simulink model "SWC_CGW_type"  (R2021b)
settings: Solver=FixedStepDiscrete  StartTime=0.0  StopTime=10.0  RelTol=1e-3
(part 3 of 3)

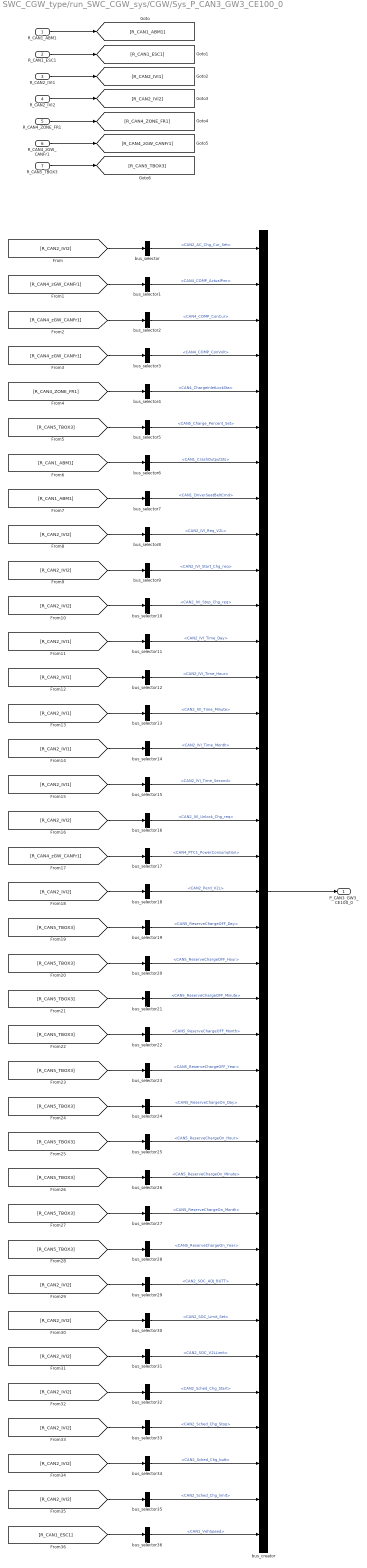
== system SWC_CGW_type/run_SWC_CGW_sys/CGW/Sys_P_CAN3_GW3_CE100_0 ==
  R_CAN1_ABM1 : Inport
  R_CAN1_ESC1 : Inport  Port=2
  R_CAN2_IVI1 : Inport  Port=3
  R_CAN2_IVI2 : Inport  Port=4
  R_CAN4_ZONE_FR1 : Inport  Port=5
  R_CAN4_zGW_CANFr1 : Inport  Port=6
  R_CAN5_TBOX3 : Inport  Port=7
  bus_creator : BusCreator  Inputs=37  OutDataTypeStr=Bus: DT_CAN3_SG_GW3_CE100_0  NonVirtualBus=on
  bus_selector : BusSelector  OutputSignals=CAN2_AC_Chg_Cur_Set
  bus_selector1 : BusSelector  OutputSignals=CAN4_COMP_ActualPwr
  bus_selector10 : BusSelector  OutputSignals=CAN2_IVI_Stop_Chg_req
  bus_selector11 : BusSelector  OutputSignals=CAN2_IVI_Time_Day
  bus_selector12 : BusSelector  OutputSignals=CAN2_IVI_Time_Hour
  bus_selector13 : BusSelector  OutputSignals=CAN2_IVI_Time_Minute
  bus_selector14 : BusSelector  OutputSignals=CAN2_IVI_Time_Month
  bus_selector15 : BusSelector  OutputSignals=CAN2_IVI_Time_Second
  bus_selector16 : BusSelector  OutputSignals=CAN2_IVI_Unlock_Chg_req
  bus_selector17 : BusSelector  OutputSignals=CAN4_PTC1_PowerConsumption
  bus_selector18 : BusSelector  OutputSignals=CAN2_Perd_V2L
  bus_selector19 : BusSelector  OutputSignals=CAN5_ReserveChargeOFF_Day
  bus_selector2 : BusSelector  OutputSignals=CAN4_COMP_ConCur
  bus_selector20 : BusSelector  OutputSignals=CAN5_ReserveChargeOFF_Hour
  bus_selector21 : BusSelector  OutputSignals=CAN5_ReserveChargeOFF_Minute
  bus_selector22 : BusSelector  OutputSignals=CAN5_ReserveChargeOFF_Month
  bus_selector23 : BusSelector  OutputSignals=CAN5_ReserveChargeOFF_Year
  bus_selector24 : BusSelector  OutputSignals=CAN5_ReserveChargeOn_Day
  bus_selector25 : BusSelector  OutputSignals=CAN5_ReserveChargeOn_Hour
  bus_selector26 : BusSelector  OutputSignals=CAN5_ReserveChargeOn_Minute
  bus_selector27 : BusSelector  OutputSignals=CAN5_ReserveChargeOn_Month
  bus_selector28 : BusSelector  OutputSignals=CAN5_ReserveChargeOn_Year
  bus_selector29 : BusSelector  OutputSignals=CAN2_SOC_ADJ_BUTT
  bus_selector3 : BusSelector  OutputSignals=CAN4_COMP_ConVolt
  bus_selector30 : BusSelector  OutputSignals=CAN2_SOC_Limit_Set
  bus_selector31 : BusSelector  OutputSignals=CAN2_SOC_V2LLimit
  bus_selector32 : BusSelector  OutputSignals=CAN2_Sched_Chg_Start
  bus_selector33 : BusSelector  OutputSignals=CAN2_Sched_Chg_Stop
  bus_selector34 : BusSelector  OutputSignals=CAN2_Sched_Chg_butt
  bus_selector35 : BusSelector  OutputSignals=CAN2_Sched_Chg_limit
  bus_selector36 : BusSelector  OutputSignals=CAN1_VehSpeed
  bus_selector4 : BusSelector  OutputSignals=CAN4_ChargeInletLockSta
  bus_selector5 : BusSelector  OutputSignals=CAN5_Charge_Percent_Set
  bus_selector6 : BusSelector  OutputSignals=CAN1_CrashOutputSts
  bus_selector7 : BusSelector  OutputSignals=CAN1_DriverSeatBeltCmd
  bus_selector8 : BusSelector  OutputSignals=CAN2_IVI_Req_V2L
  bus_selector9 : BusSelector  OutputSignals=CAN2_IVI_Start_Chg_req
  P_CAN3_GW3_CE100_0 : Outport
  wires:
  bus_creator/1 -> P_CAN3_GW3_CE100_0/1
  bus_selector/1 -> bus_creator/1  "<CAN2_AC_Chg_Cur_Set>"
  [R_CAN2_IVI2] -> bus_selector/1
  bus_selector1/1 -> bus_creator/2  "<CAN4_COMP_ActualPwr>"
  [R_CAN4_zGW_CANFr1] -> bus_selector1/1
  bus_selector2/1 -> bus_creator/3  "<CAN4_COMP_ConCur>"
  [R_CAN4_zGW_CANFr1] -> bus_selector2/1
  bus_selector3/1 -> bus_creator/4  "<CAN4_COMP_ConVolt>"
  [R_CAN4_zGW_CANFr1] -> bus_selector3/1
  bus_selector4/1 -> bus_creator/5  "<CAN4_ChargeInletLockSta>"
  [R_CAN4_ZONE_FR1] -> bus_selector4/1
  bus_selector5/1 -> bus_creator/6  "<CAN5_Charge_Percent_Set>"
  [R_CAN5_TBOX3] -> bus_selector5/1
  bus_selector6/1 -> bus_creator/7  "<CAN1_CrashOutputSts>"
  [R_CAN1_ABM1] -> bus_selector6/1
  bus_selector7/1 -> bus_creator/8  "<CAN1_DriverSeatBeltCmd>"
  [R_CAN1_ABM1] -> bus_selector7/1
  bus_selector8/1 -> bus_creator/9  "<CAN2_IVI_Req_V2L>"
  [R_CAN2_IVI2] -> bus_selector8/1
  bus_selector9/1 -> bus_creator/10  "<CAN2_IVI_Start_Chg_req>"
  [R_CAN2_IVI2] -> bus_selector9/1
  bus_selector10/1 -> bus_creator/11  "<CAN2_IVI_Stop_Chg_req>"
  [R_CAN2_IVI2] -> bus_selector10/1
  bus_selector11/1 -> bus_creator/12  "<CAN2_IVI_Time_Day>"
  [R_CAN2_IVI1] -> bus_selector11/1
  bus_selector12/1 -> bus_creator/13  "<CAN2_IVI_Time_Hour>"
  [R_CAN2_IVI1] -> bus_selector12/1
  bus_selector13/1 -> bus_creator/14  "<CAN2_IVI_Time_Minute>"
  [R_CAN2_IVI1] -> bus_selector13/1
  bus_selector14/1 -> bus_creator/15  "<CAN2_IVI_Time_Month>"
  [R_CAN2_IVI1] -> bus_selector14/1
  bus_selector15/1 -> bus_creator/16  "<CAN2_IVI_Time_Second>"
  [R_CAN2_IVI1] -> bus_selector15/1
  bus_selector16/1 -> bus_creator/17  "<CAN2_IVI_Unlock_Chg_req>"
  [R_CAN2_IVI2] -> bus_selector16/1
  bus_selector17/1 -> bus_creator/18  "<CAN4_PTC1_PowerConsumption>"
  [R_CAN4_zGW_CANFr1] -> bus_selector17/1
  bus_selector18/1 -> bus_creator/19  "<CAN2_Perd_V2L>"
  [R_CAN2_IVI2] -> bus_selector18/1
  bus_selector19/1 -> bus_creator/20  "<CAN5_ReserveChargeOFF_Day>"
  [R_CAN5_TBOX3] -> bus_selector19/1
  bus_selector20/1 -> bus_creator/21  "<CAN5_ReserveChargeOFF_Hour>"
  [R_CAN5_TBOX3] -> bus_selector20/1
  bus_selector21/1 -> bus_creator/22  "<CAN5_ReserveChargeOFF_Minute>"
  [R_CAN5_TBOX3] -> bus_selector21/1
  bus_selector22/1 -> bus_creator/23  "<CAN5_ReserveChargeOFF_Month>"
  [R_CAN5_TBOX3] -> bus_selector22/1
  bus_selector23/1 -> bus_creator/24  "<CAN5_ReserveChargeOFF_Year>"
  [R_CAN5_TBOX3] -> bus_selector23/1
  bus_selector24/1 -> bus_creator/25  "<CAN5_ReserveChargeOn_Day>"
  [R_CAN5_TBOX3] -> bus_selector24/1
  bus_selector25/1 -> bus_creator/26  "<CAN5_ReserveChargeOn_Hour>"
  [R_CAN5_TBOX3] -> bus_selector25/1
  bus_selector26/1 -> bus_creator/27  "<CAN5_ReserveChargeOn_Minute>"
  [R_CAN5_TBOX3] -> bus_selector26/1
  bus_selector27/1 -> bus_creator/28  "<CAN5_ReserveChargeOn_Month>"
  [R_CAN5_TBOX3] -> bus_selector27/1
  bus_selector28/1 -> bus_creator/29  "<CAN5_ReserveChargeOn_Year>"
  [R_CAN5_TBOX3] -> bus_selector28/1
  bus_selector29/1 -> bus_creator/30  "<CAN2_SOC_ADJ_BUTT>"
  [R_CAN2_IVI2] -> bus_selector29/1
  bus_selector30/1 -> bus_creator/31  "<CAN2_SOC_Limit_Set>"
  [R_CAN2_IVI2] -> bus_selector30/1
  bus_selector31/1 -> bus_creator/32  "<CAN2_SOC_V2LLimit>"
  [R_CAN2_IVI2] -> bus_selector31/1
  bus_selector32/1 -> bus_creator/33  "<CAN2_Sched_Chg_Start>"
  [R_CAN2_IVI2] -> bus_selector32/1
  bus_selector33/1 -> bus_creator/34  "<CAN2_Sched_Chg_Stop>"
  [R_CAN2_IVI2] -> bus_selector33/1
  bus_selector34/1 -> bus_creator/35  "<CAN2_Sched_Chg_butt>"
  [R_CAN2_IVI2] -> bus_selector34/1
  bus_selector35/1 -> bus_creator/36  "<CAN2_Sched_Chg_limit>"
  [R_CAN2_IVI2] -> bus_selector35/1
  bus_selector36/1 -> bus_creator/37  "<CAN1_VehSpeed>"
  [R_CAN1_ESC1] -> bus_selector36/1
  R_CAN1_ABM1/1 -> [R_CAN1_ABM1]
  R_CAN1_ESC1/1 -> [R_CAN1_ESC1]
  R_CAN2_IVI1/1 -> [R_CAN2_IVI1]
  R_CAN2_IVI2/1 -> [R_CAN2_IVI2]
  R_CAN4_ZONE_FR1/1 -> [R_CAN4_ZONE_FR1]
  R_CAN4_zGW_CANFr1/1 -> [R_CAN4_zGW_CANFr1]
  R_CAN5_TBOX3/1 -> [R_CAN5_TBOX3]

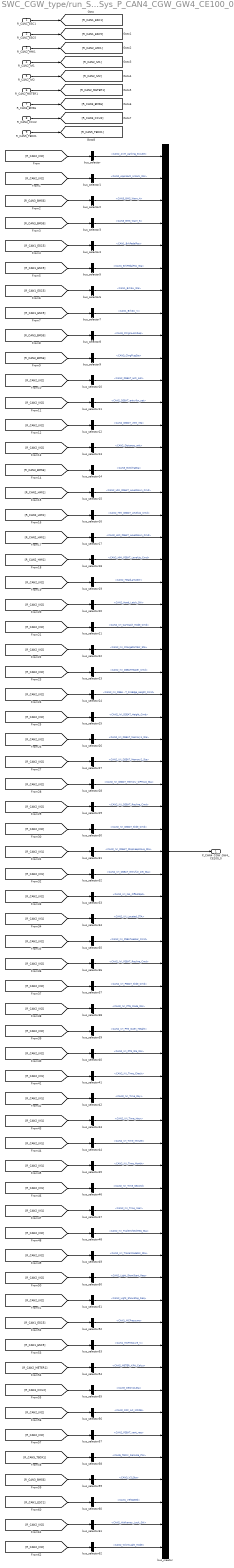
== system SWC_CGW_type/run_SWC_CGW_sys/CGW/Sys_P_CAN4_CGW_GW4_CE100_0 ==
  R_CAN1_ESC1 : Inport
  R_CAN1_ESC5 : Inport  Port=2
  R_CAN2_HMI1 : Inport  Port=3
  R_CAN2_IVI1 : Inport  Port=4
  R_CAN2_IVI2 : Inport  Port=5
  R_CAN2_METER1 : Inport  Port=6
  R_CAN3_BMS6 : Inport  Port=7
  R_CAN3_CCU2 : Inport  Port=8
  R_CAN5_TBOX1 : Inport  Port=9
  bus_creator : BusCreator  Inputs=63  OutDataTypeStr=Bus: DT_CAN4_SG_CGW_GW4_CE100_0  NonVirtualBus=on
  bus_selector : BusSelector  OutputSignals=CAN2_AVM_parking_excute
  bus_selector1 : BusSelector  OutputSignals=CAN2_Approach_Unlock_SW
  bus_selector10 : BusSelector  OutputSignals=CAN2_DSEAT_anti_set
  bus_selector11 : BusSelector  OutputSignals=CAN2_DSEAT_entryfun_set
  bus_selector12 : BusSelector  OutputSignals=CAN2_DSEAT_vent_req
  bus_selector13 : BusSelector  OutputSignals=CAN2_Distance_unit
  bus_selector14 : BusSelector  OutputSignals=CAN3_ExtChrgSta
  bus_selector15 : BusSelector  OutputSignals=CAN2_HMI_DSEAT_LevelDown_Cmd
  bus_selector16 : BusSelector  OutputSignals=CAN2_HMI_DSEAT_LevelUp_Cmd
  bus_selector17 : BusSelector  OutputSignals=CAN2_HMI_PSEAT_LevelDown_Cmd
  bus_selector18 : BusSelector  OutputSignals=CAN2_HMI_PSEAT_LevelUp_Cmd
  bus_selector19 : BusSelector  OutputSignals=CAN2_HeadLampSW
  bus_selector2 : BusSelector  OutputSignals=CAN3_BMS_Warn_4
  bus_selector20 : BusSelector  OutputSignals=CAN2_Hood_Latch_SW
  bus_selector21 : BusSelector  OutputSignals=CAN2_IVI_CarWash_Mode_Cmd
  bus_selector22 : BusSelector  OutputSignals=CAN2_IVI_ChargePortSW_Sta
  bus_selector23 : BusSelector  OutputSignals=CAN2_IVI_DSEATHeater_Cmd
  bus_selector24 : BusSelector  OutputSignals=CAN2_IVI_DSEAT_FroEdge_Height_Cmd
  bus_selector25 : BusSelector  OutputSignals=CAN2_IVI_DSEAT_Height_Cmd
  bus_selector26 : BusSelector  OutputSignals=CAN2_IVI_DSEAT_Memory1_Sta
  bus_selector27 : BusSelector  OutputSignals=CAN2_IVI_DSEAT_Memory2_Sta
  bus_selector28 : BusSelector  OutputSignals=CAN2_IVI_DSEAT_Memory_OPTCLS_Sta
  bus_selector29 : BusSelector  OutputSignals=CAN2_IVI_DSEAT_Recline_Cmd
  bus_selector3 : BusSelector  OutputSignals=CAN3_BMS_Warn_5
  bus_selector30 : BusSelector  OutputSignals=CAN2_IVI_DSEAT_Slide_Cmd
  bus_selector31 : BusSelector  OutputSignals=CAN2_IVI_DSEAT_StopKeepMove_Sta
  bus_selector32 : BusSelector  OutputSignals=CAN2_IVI_DSEAT_entryfun_set_Sta
  bus_selector33 : BusSelector  OutputSignals=CAN2_IVI_ISA_OffsetSpd
  bus_selector34 : BusSelector  OutputSignals=CAN2_IVI_Located_STA
  bus_selector35 : BusSelector  OutputSignals=CAN2_IVI_PSEATHeater_Cmd
  bus_selector36 : BusSelector  OutputSignals=CAN2_IVI_PSEAT_Recline_Cmd
  bus_selector37 : BusSelector  OutputSignals=CAN2_IVI_PSEAT_Slide_Cmd
  bus_selector38 : BusSelector  OutputSignals=CAN2_IVI_PTG_Mode_SW
  bus_selector39 : BusSelector  OutputSignals=CAN2_IVI_PTG_Open_Height
  bus_selector4 : BusSelector  OutputSignals=CAN1_BrkPedalPos
  bus_selector40 : BusSelector  OutputSignals=CAN2_IVI_PTG_Sta_SW
  bus_selector41 : BusSelector  OutputSignals=CAN2_IVI_Time_Check
  bus_selector42 : BusSelector  OutputSignals=CAN2_IVI_Time_Day
  bus_selector43 : BusSelector  OutputSignals=CAN2_IVI_Time_Hour
  bus_selector44 : BusSelector  OutputSignals=CAN2_IVI_Time_Minute
  bus_selector45 : BusSelector  OutputSignals=CAN2_IVI_Time_Month
  bus_selector46 : BusSelector  OutputSignals=CAN2_IVI_Time_Second
  bus_selector47 : BusSelector  OutputSignals=CAN2_IVI_Time_Year
  bus_selector48 : BusSelector  OutputSignals=CAN2_IVI_TrailerCheckReq_Sta
  bus_selector49 : BusSelector  OutputSignals=CAN2_IVI_TrailerModeSW_Sta
  bus_selector5 : BusSelector  OutputSignals=CAN1_BrkPedalPos_Sta
  bus_selector50 : BusSelector  OutputSignals=CAN2_Light_ShowStart_Req
  bus_selector51 : BusSelector  OutputSignals=CAN2_Light_ShowStop_Req
  bus_selector52 : BusSelector  OutputSignals=CAN1_MCPressure
  bus_selector53 : BusSelector  OutputSignals=CAN1_MCPressure_V
  bus_selector54 : BusSelector  OutputSignals=CAN2_METER_KPH_Calcu
  bus_selector55 : BusSelector  OutputSignals=CAN3_OBCV2LSta
  bus_selector56 : BusSelector  OutputSignals=CAN2_OFF_AC_MODE
  bus_selector57 : BusSelector  OutputSignals=CAN2_PSEAT_vent_req
  bus_selector58 : BusSelector  OutputSignals=CAN5_TBOX_Remote_PW
  bus_selector59 : BusSelector  OutputSignals=CAN3_V2LSta
  bus_selector6 : BusSelector  OutputSignals=CAN1_BrkSw_Sta
  bus_selector60 : BusSelector  OutputSignals=CAN1_VehSpeed
  bus_selector61 : BusSelector  OutputSignals=CAN2_Walkaway_Lock_SW
  bus_selector62 : BusSelector  OutputSignals=CAN2_WlcmLight_Mode
  bus_selector7 : BusSelector  OutputSignals=CAN1_BrkSw_V
  bus_selector8 : BusSelector  OutputSignals=CAN3_ChrgInLockReq
  bus_selector9 : BusSelector  OutputSignals=CAN3_ChrgPlugSta
  P_CAN4_CGW_GW4_CE100_0 : Outport
  wires:
  bus_creator/1 -> P_CAN4_CGW_GW4_CE100_0/1
  bus_selector/1 -> bus_creator/1  "<CAN2_AVM_parking_excute>"
  [R_CAN2_IVI2] -> bus_selector/1
  bus_selector1/1 -> bus_creator/2  "<CAN2_Approach_Unlock_SW>"
  [R_CAN2_IVI2] -> bus_selector1/1
  bus_selector2/1 -> bus_creator/3  "<CAN3_BMS_Warn_4>"
  [R_CAN3_BMS6] -> bus_selector2/1
  bus_selector3/1 -> bus_creator/4  "<CAN3_BMS_Warn_5>"
  [R_CAN3_BMS6] -> bus_selector3/1
  bus_selector4/1 -> bus_creator/5  "<CAN1_BrkPedalPos>"
  [R_CAN1_ESC5] -> bus_selector4/1
  bus_selector5/1 -> bus_creator/6  "<CAN1_BrkPedalPos_Sta>"
  [R_CAN1_ESC5] -> bus_selector5/1
  bus_selector6/1 -> bus_creator/7  "<CAN1_BrkSw_Sta>"
  [R_CAN1_ESC5] -> bus_selector6/1
  bus_selector7/1 -> bus_creator/8  "<CAN1_BrkSw_V>"
  [R_CAN1_ESC5] -> bus_selector7/1
  bus_selector8/1 -> bus_creator/9  "<CAN3_ChrgInLockReq>"
  [R_CAN3_BMS6] -> bus_selector8/1
  bus_selector9/1 -> bus_creator/10  "<CAN3_ChrgPlugSta>"
  [R_CAN3_BMS6] -> bus_selector9/1
  bus_selector10/1 -> bus_creator/11  "<CAN2_DSEAT_anti_set>"
  [R_CAN2_IVI2] -> bus_selector10/1
  bus_selector11/1 -> bus_creator/12  "<CAN2_DSEAT_entryfun_set>"
  [R_CAN2_IVI2] -> bus_selector11/1
  bus_selector12/1 -> bus_creator/13  "<CAN2_DSEAT_vent_req>"
  [R_CAN2_IVI2] -> bus_selector12/1
  bus_selector13/1 -> bus_creator/14  "<CAN2_Distance_unit>"
  [R_CAN2_IVI2] -> bus_selector13/1
  bus_selector14/1 -> bus_creator/15  "<CAN3_ExtChrgSta>"
  [R_CAN3_BMS6] -> bus_selector14/1
  bus_selector15/1 -> bus_creator/16  "<CAN2_HMI_DSEAT_LevelDown_Cmd>"
  [R_CAN2_HMI1] -> bus_selector15/1
  bus_selector16/1 -> bus_creator/17  "<CAN2_HMI_DSEAT_LevelUp_Cmd>"
  [R_CAN2_HMI1] -> bus_selector16/1
  bus_selector17/1 -> bus_creator/18  "<CAN2_HMI_PSEAT_LevelDown_Cmd>"
  [R_CAN2_HMI1] -> bus_selector17/1
  bus_selector18/1 -> bus_creator/19  "<CAN2_HMI_PSEAT_LevelUp_Cmd>"
  [R_CAN2_HMI1] -> bus_selector18/1
  bus_selector19/1 -> bus_creator/20  "<CAN2_HeadLampSW>"
  [R_CAN2_IVI2] -> bus_selector19/1
  bus_selector20/1 -> bus_creator/21  "<CAN2_Hood_Latch_SW>"
  [R_CAN2_IVI2] -> bus_selector20/1
  bus_selector21/1 -> bus_creator/22  "<CAN2_IVI_CarWash_Mode_Cmd>"
  [R_CAN2_IVI2] -> bus_selector21/1
  bus_selector22/1 -> bus_creator/23  "<CAN2_IVI_ChargePortSW_Sta>"
  [R_CAN2_IVI2] -> bus_selector22/1
  bus_selector23/1 -> bus_creator/24  "<CAN2_IVI_DSEATHeater_Cmd>"
  [R_CAN2_IVI2] -> bus_selector23/1
  bus_selector24/1 -> bus_creator/25  "<CAN2_IVI_DSEAT_FroEdge_Height_Cmd>"
  [R_CAN2_IVI2] -> bus_selector24/1
  bus_selector25/1 -> bus_creator/26  "<CAN2_IVI_DSEAT_Height_Cmd>"
  [R_CAN2_IVI2] -> bus_selector25/1
  bus_selector26/1 -> bus_creator/27  "<CAN2_IVI_DSEAT_Memory1_Sta>"
  [R_CAN2_IVI2] -> bus_selector26/1
  bus_selector27/1 -> bus_creator/28  "<CAN2_IVI_DSEAT_Memory2_Sta>"
  [R_CAN2_IVI2] -> bus_selector27/1
  bus_selector28/1 -> bus_creator/29  "<CAN2_IVI_DSEAT_Memory_OPTCLS_Sta>"
  [R_CAN2_IVI2] -> bus_selector28/1
  bus_selector29/1 -> bus_creator/30  "<CAN2_IVI_DSEAT_Recline_Cmd>"
  [R_CAN2_IVI2] -> bus_selector29/1
  bus_selector30/1 -> bus_creator/31  "<CAN2_IVI_DSEAT_Slide_Cmd>"
  [R_CAN2_IVI2] -> bus_selector30/1
  bus_selector31/1 -> bus_creator/32  "<CAN2_IVI_DSEAT_StopKeepMove_Sta>"
  [R_CAN2_IVI1] -> bus_selector31/1
  bus_selector32/1 -> bus_creator/33  "<CAN2_IVI_DSEAT_entryfun_set_Sta>"
  [R_CAN2_IVI1] -> bus_selector32/1
  bus_selector33/1 -> bus_creator/34  "<CAN2_IVI_ISA_OffsetSpd>"
  [R_CAN2_IVI2] -> bus_selector33/1
  bus_selector34/1 -> bus_creator/35  "<CAN2_IVI_Located_STA>"
  [R_CAN2_IVI1] -> bus_selector34/1
  bus_selector35/1 -> bus_creator/36  "<CAN2_IVI_PSEATHeater_Cmd>"
  [R_CAN2_IVI2] -> bus_selector35/1
  bus_selector36/1 -> bus_creator/37  "<CAN2_IVI_PSEAT_Recline_Cmd>"
  [R_CAN2_IVI2] -> bus_selector36/1
  bus_selector37/1 -> bus_creator/38  "<CAN2_IVI_PSEAT_Slide_Cmd>"
  [R_CAN2_IVI2] -> bus_selector37/1
  bus_selector38/1 -> bus_creator/39  "<CAN2_IVI_PTG_Mode_SW>"
  [R_CAN2_IVI2] -> bus_selector38/1
  bus_selector39/1 -> bus_creator/40  "<CAN2_IVI_PTG_Open_Height>"
  [R_CAN2_IVI2] -> bus_selector39/1
  bus_selector40/1 -> bus_creator/41  "<CAN2_IVI_PTG_Sta_SW>"
  [R_CAN2_IVI2] -> bus_selector40/1
  bus_selector41/1 -> bus_creator/42  "<CAN2_IVI_Time_Check>"
  [R_CAN2_IVI1] -> bus_selector41/1
  bus_selector42/1 -> bus_creator/43  "<CAN2_IVI_Time_Day>"
  [R_CAN2_IVI1] -> bus_selector42/1
  bus_selector43/1 -> bus_creator/44  "<CAN2_IVI_Time_Hour>"
  [R_CAN2_IVI1] -> bus_selector43/1
  bus_selector44/1 -> bus_creator/45  "<CAN2_IVI_Time_Minute>"
  [R_CAN2_IVI1] -> bus_selector44/1
  bus_selector45/1 -> bus_creator/46  "<CAN2_IVI_Time_Month>"
  [R_CAN2_IVI1] -> bus_selector45/1
  bus_selector46/1 -> bus_creator/47  "<CAN2_IVI_Time_Second>"
  [R_CAN2_IVI1] -> bus_selector46/1
  bus_selector47/1 -> bus_creator/48  "<CAN2_IVI_Time_Year>"
  [R_CAN2_IVI1] -> bus_selector47/1
  bus_selector48/1 -> bus_creator/49  "<CAN2_IVI_TrailerCheckReq_Sta>"
  [R_CAN2_IVI2] -> bus_selector48/1
  bus_selector49/1 -> bus_creator/50  "<CAN2_IVI_TrailerModeSW_Sta>"
  [R_CAN2_IVI2] -> bus_selector49/1
  bus_selector50/1 -> bus_creator/51  "<CAN2_Light_ShowStart_Req>"
  [R_CAN2_IVI2] -> bus_selector50/1
  bus_selector51/1 -> bus_creator/52  "<CAN2_Light_ShowStop_Req>"
  [R_CAN2_IVI2] -> bus_selector51/1
  bus_selector52/1 -> bus_creator/53  "<CAN1_MCPressure>"
  [R_CAN1_ESC5] -> bus_selector52/1
  bus_selector53/1 -> bus_creator/54  "<CAN1_MCPressure_V>"
  [R_CAN1_ESC5] -> bus_selector53/1
  bus_selector54/1 -> bus_creator/55  "<CAN2_METER_KPH_Calcu>"
  [R_CAN2_METER1] -> bus_selector54/1
  bus_selector55/1 -> bus_creator/56  "<CAN3_OBCV2LSta>"
  [R_CAN3_CCU2] -> bus_selector55/1
  bus_selector56/1 -> bus_creator/57  "<CAN2_OFF_AC_MODE>"
  [R_CAN2_IVI2] -> bus_selector56/1
  bus_selector57/1 -> bus_creator/58  "<CAN2_PSEAT_vent_req>"
  [R_CAN2_IVI2] -> bus_selector57/1
  bus_selector58/1 -> bus_creator/59  "<CAN5_TBOX_Remote_PW>"
  [R_CAN5_TBOX1] -> bus_selector58/1
  bus_selector59/1 -> bus_creator/60  "<CAN3_V2LSta>"
  [R_CAN3_BMS6] -> bus_selector59/1
  bus_selector60/1 -> bus_creator/61  "<CAN1_VehSpeed>"
  [R_CAN1_ESC1] -> bus_selector60/1
  bus_selector61/1 -> bus_creator/62  "<CAN2_Walkaway_Lock_SW>"
  [R_CAN2_IVI2] -> bus_selector61/1
  bus_selector62/1 -> bus_creator/63  "<CAN2_WlcmLight_Mode>"
  [R_CAN2_IVI2] -> bus_selector62/1
  R_CAN1_ESC1/1 -> [R_CAN1_ESC1]
  R_CAN1_ESC5/1 -> [R_CAN1_ESC5]
  R_CAN2_HMI1/1 -> [R_CAN2_HMI1]
  R_CAN2_IVI1/1 -> [R_CAN2_IVI1]
  R_CAN2_IVI2/1 -> [R_CAN2_IVI2]
  R_CAN2_METER1/1 -> [R_CAN2_METER1]
  R_CAN3_BMS6/1 -> [R_CAN3_BMS6]
  R_CAN3_CCU2/1 -> [R_CAN3_CCU2]
  R_CAN5_TBOX1/1 -> [R_CAN5_TBOX1]

== system SWC_CGW_type/run_SWC_CGW_sys/CGW/Sys_P_CAN4_GW4_CE200_0 ==
  R_CAN2_IVI3 : Inport
  bus_creator : BusCreator  Inputs=22  OutDataTypeStr=Bus: DT_CAN4_SG_GW4_CE200_0  NonVirtualBus=on
  bus_selector : BusSelector  OutputSignals=CAN2_IVI_LSEATvent_Cmd
  bus_selector1 : BusSelector  OutputSignals=CAN2_IVI_MLFMost_Cmd
  bus_selector10 : BusSelector  OutputSignals=CAN2_IVI_MLZeroGravity_Cmd
  bus_selector11 : BusSelector  OutputSignals=CAN2_IVI_MRFMost_Cmd
  bus_selector12 : BusSelector  OutputSignals=CAN2_IVI_MRFootLift_Cmd
  bus_selector13 : BusSelector  OutputSignals=CAN2_IVI_MRNapMode_Cmd
  bus_selector14 : BusSelector  OutputSignals=CAN2_IVI_MRRecliner_Cmd
  bus_selector15 : BusSelector  OutputSignals=CAN2_IVI_MRRestore_Cmd
  bus_selector16 : BusSelector  OutputSignals=CAN2_IVI_MRSEATvent_Cmd
  bus_selector17 : BusSelector  OutputSignals=CAN2_IVI_MRSeatLift_Cmd
  bus_selector18 : BusSelector  OutputSignals=CAN2_IVI_MRSldRestore_Cmd
  bus_selector19 : BusSelector  OutputSignals=CAN2_IVI_MRSlider_Cmd
  bus_selector2 : BusSelector  OutputSignals=CAN2_IVI_MLFootLift_Cmd
  bus_selector20 : BusSelector  OutputSignals=CAN2_IVI_MRZeroGravity_Cmd
  bus_selector21 : BusSelector  OutputSignals=CAN2_IVI_RSEATvent_Cmd
  bus_selector3 : BusSelector  OutputSignals=CAN2_IVI_MLNapMode_Cmd
  bus_selector4 : BusSelector  OutputSignals=CAN2_IVI_MLRecliner_Cmd
  bus_selector5 : BusSelector  OutputSignals=CAN2_IVI_MLRestore_Cmd
  bus_selector6 : BusSelector  OutputSignals=CAN2_IVI_MLSEATvent_Cmd
  bus_selector7 : BusSelector  OutputSignals=CAN2_IVI_MLSeatLift_Cmd
  bus_selector8 : BusSelector  OutputSignals=CAN2_IVI_MLSldRestore_Cmd
  bus_selector9 : BusSelector  OutputSignals=CAN2_IVI_MLSlider_Cmd
  P_CAN4_GW4_CE200_0 : Outport
  wires:
  bus_creator/1 -> P_CAN4_GW4_CE200_0/1
  bus_selector/1 -> bus_creator/1  "<CAN2_IVI_LSEATvent_Cmd>"
  [R_CAN2_IVI3] -> bus_selector/1
  bus_selector1/1 -> bus_creator/2  "<CAN2_IVI_MLFMost_Cmd>"
  [R_CAN2_IVI3] -> bus_selector1/1
  bus_selector2/1 -> bus_creator/3  "<CAN2_IVI_MLFootLift_Cmd>"
  [R_CAN2_IVI3] -> bus_selector2/1
  bus_selector3/1 -> bus_creator/4  "<CAN2_IVI_MLNapMode_Cmd>"
  [R_CAN2_IVI3] -> bus_selector3/1
  bus_selector4/1 -> bus_creator/5  "<CAN2_IVI_MLRecliner_Cmd>"
  [R_CAN2_IVI3] -> bus_selector4/1
  bus_selector5/1 -> bus_creator/6  "<CAN2_IVI_MLRestore_Cmd>"
  [R_CAN2_IVI3] -> bus_selector5/1
  bus_selector6/1 -> bus_creator/7  "<CAN2_IVI_MLSEATvent_Cmd>"
  [R_CAN2_IVI3] -> bus_selector6/1
  bus_selector7/1 -> bus_creator/8  "<CAN2_IVI_MLSeatLift_Cmd>"
  [R_CAN2_IVI3] -> bus_selector7/1
  bus_selector8/1 -> bus_creator/9  "<CAN2_IVI_MLSldRestore_Cmd>"
  [R_CAN2_IVI3] -> bus_selector8/1
  bus_selector9/1 -> bus_creator/10  "<CAN2_IVI_MLSlider_Cmd>"
  [R_CAN2_IVI3] -> bus_selector9/1
  bus_selector10/1 -> bus_creator/11  "<CAN2_IVI_MLZeroGravity_Cmd>"
  [R_CAN2_IVI3] -> bus_selector10/1
  bus_selector11/1 -> bus_creator/12  "<CAN2_IVI_MRFMost_Cmd>"
  [R_CAN2_IVI3] -> bus_selector11/1
  bus_selector12/1 -> bus_creator/13  "<CAN2_IVI_MRFootLift_Cmd>"
  [R_CAN2_IVI3] -> bus_selector12/1
  bus_selector13/1 -> bus_creator/14  "<CAN2_IVI_MRNapMode_Cmd>"
  [R_CAN2_IVI3] -> bus_selector13/1
  bus_selector14/1 -> bus_creator/15  "<CAN2_IVI_MRRecliner_Cmd>"
  [R_CAN2_IVI3] -> bus_selector14/1
  bus_selector15/1 -> bus_creator/16  "<CAN2_IVI_MRRestore_Cmd>"
  [R_CAN2_IVI3] -> bus_selector15/1
  bus_selector16/1 -> bus_creator/17  "<CAN2_IVI_MRSEATvent_Cmd>"
  [R_CAN2_IVI3] -> bus_selector16/1
  bus_selector17/1 -> bus_creator/18  "<CAN2_IVI_MRSeatLift_Cmd>"
  [R_CAN2_IVI3] -> bus_selector17/1
  bus_selector18/1 -> bus_creator/19  "<CAN2_IVI_MRSldRestore_Cmd>"
  [R_CAN2_IVI3] -> bus_selector18/1
  bus_selector19/1 -> bus_creator/20  "<CAN2_IVI_MRSlider_Cmd>"
  [R_CAN2_IVI3] -> bus_selector19/1
  bus_selector20/1 -> bus_creator/21  "<CAN2_IVI_MRZeroGravity_Cmd>"
  [R_CAN2_IVI3] -> bus_selector20/1
  bus_selector21/1 -> bus_creator/22  "<CAN2_IVI_RSEATvent_Cmd>"
  [R_CAN2_IVI3] -> bus_selector21/1
  R_CAN2_IVI3/1 -> [R_CAN2_IVI3]

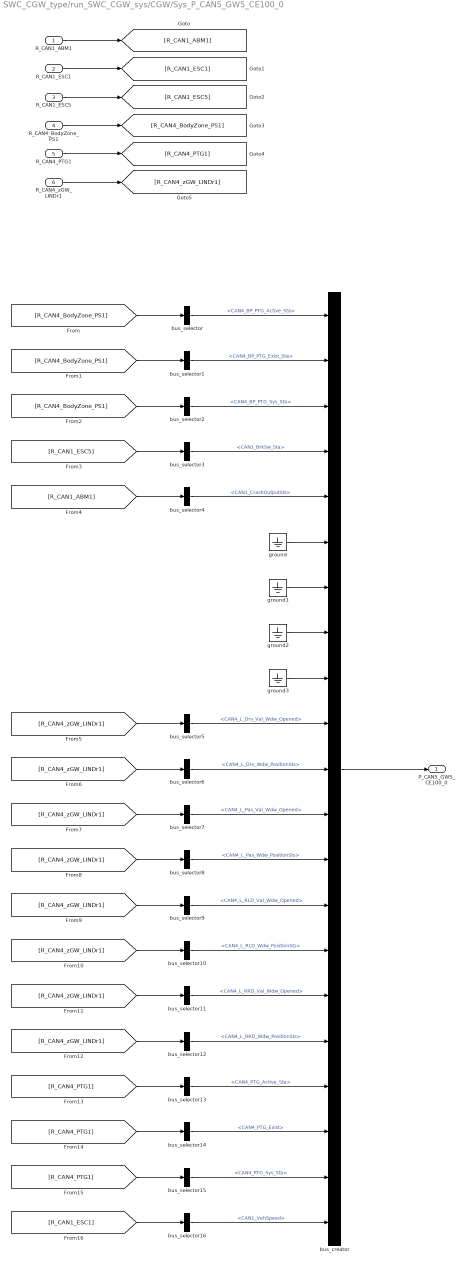
== system SWC_CGW_type/run_SWC_CGW_sys/CGW/Sys_P_CAN5_GW5_CE100_0 ==
  R_CAN1_ABM1 : Inport
  R_CAN1_ESC1 : Inport  Port=2
  R_CAN1_ESC5 : Inport  Port=3
  R_CAN4_BodyZone_PS1 : Inport  Port=4
  R_CAN4_PTG1 : Inport  Port=5
  R_CAN4_zGW_LINDr1 : Inport  Port=6
  bus_creator : BusCreator  Inputs=21  OutDataTypeStr=Bus: DT_CAN5_SG_GW5_CE100_0  NonVirtualBus=on
  bus_selector : BusSelector  OutputSignals=CAN4_BP_PTG_Active_Sta
  bus_selector1 : BusSelector  OutputSignals=CAN4_BP_PTG_Exist_Sta
  bus_selector10 : BusSelector  OutputSignals=CAN4_L_RLD_Wdw_PositionSts
  bus_selector11 : BusSelector  OutputSignals=CAN4_L_RRD_Val_Wdw_Opened
  bus_selector12 : BusSelector  OutputSignals=CAN4_L_RRD_Wdw_PositionSts
  bus_selector13 : BusSelector  OutputSignals=CAN4_PTG_Active_Sta
  bus_selector14 : BusSelector  OutputSignals=CAN4_PTG_Exist
  bus_selector15 : BusSelector  OutputSignals=CAN4_PTG_Sys_Sta
  bus_selector16 : BusSelector  OutputSignals=CAN1_VehSpeed
  bus_selector2 : BusSelector  OutputSignals=CAN4_BP_PTG_Sys_Sta
  bus_selector3 : BusSelector  OutputSignals=CAN1_BrkSw_Sta
  bus_selector4 : BusSelector  OutputSignals=CAN1_CrashOutputSts
  bus_selector5 : BusSelector  OutputSignals=CAN4_L_Drv_Val_Wdw_Opened
  bus_selector6 : BusSelector  OutputSignals=CAN4_L_Drv_Wdw_PositionSts
  bus_selector7 : BusSelector  OutputSignals=CAN4_L_Pas_Val_Wdw_Opened
  bus_selector8 : BusSelector  OutputSignals=CAN4_L_Pas_Wdw_PositionSts
  bus_selector9 : BusSelector  OutputSignals=CAN4_L_RLD_Val_Wdw_Opened
  ground{,1..3} (4 alike) : Ground
  P_CAN5_GW5_CE100_0 : Outport
  wires:
  bus_creator/1 -> P_CAN5_GW5_CE100_0/1
  bus_selector/1 -> bus_creator/1  "<CAN4_BP_PTG_Active_Sta>"
  [R_CAN4_BodyZone_PS1] -> bus_selector/1
  bus_selector1/1 -> bus_creator/2  "<CAN4_BP_PTG_Exist_Sta>"
  [R_CAN4_BodyZone_PS1] -> bus_selector1/1
  bus_selector2/1 -> bus_creator/3  "<CAN4_BP_PTG_Sys_Sta>"
  [R_CAN4_BodyZone_PS1] -> bus_selector2/1
  bus_selector3/1 -> bus_creator/4  "<CAN1_BrkSw_Sta>"
  [R_CAN1_ESC5] -> bus_selector3/1
  bus_selector4/1 -> bus_creator/5  "<CAN1_CrashOutputSts>"
  [R_CAN1_ABM1] -> bus_selector4/1
  ground/1 -> bus_creator/6
  ground1/1 -> bus_creator/7
  ground2/1 -> bus_creator/8
  ground3/1 -> bus_creator/9
  bus_selector5/1 -> bus_creator/10  "<CAN4_L_Drv_Val_Wdw_Opened>"
  [R_CAN4_zGW_LINDr1] -> bus_selector5/1
  bus_selector6/1 -> bus_creator/11  "<CAN4_L_Drv_Wdw_PositionSts>"
  [R_CAN4_zGW_LINDr1] -> bus_selector6/1
  bus_selector7/1 -> bus_creator/12  "<CAN4_L_Pas_Val_Wdw_Opened>"
  [R_CAN4_zGW_LINDr1] -> bus_selector7/1
  bus_selector8/1 -> bus_creator/13  "<CAN4_L_Pas_Wdw_PositionSts>"
  [R_CAN4_zGW_LINDr1] -> bus_selector8/1
  bus_selector9/1 -> bus_creator/14  "<CAN4_L_RLD_Val_Wdw_Opened>"
  [R_CAN4_zGW_LINDr1] -> bus_selector9/1
  bus_selector10/1 -> bus_creator/15  "<CAN4_L_RLD_Wdw_PositionSts>"
  [R_CAN4_zGW_LINDr1] -> bus_selector10/1
  bus_selector11/1 -> bus_creator/16  "<CAN4_L_RRD_Val_Wdw_Opened>"
  [R_CAN4_zGW_LINDr1] -> bus_selector11/1
  bus_selector12/1 -> bus_creator/17  "<CAN4_L_RRD_Wdw_PositionSts>"
  [R_CAN4_zGW_LINDr1] -> bus_selector12/1
  bus_selector13/1 -> bus_creator/18  "<CAN4_PTG_Active_Sta>"
  [R_CAN4_PTG1] -> bus_selector13/1
  bus_selector14/1 -> bus_creator/19  "<CAN4_PTG_Exist>"
  [R_CAN4_PTG1] -> bus_selector14/1
  bus_selector15/1 -> bus_creator/20  "<CAN4_PTG_Sys_Sta>"
  [R_CAN4_PTG1] -> bus_selector15/1
  bus_selector16/1 -> bus_creator/21  "<CAN1_VehSpeed>"
  [R_CAN1_ESC1] -> bus_selector16/1
  R_CAN1_ABM1/1 -> [R_CAN1_ABM1]
  R_CAN1_ESC1/1 -> [R_CAN1_ESC1]
  R_CAN1_ESC5/1 -> [R_CAN1_ESC5]
  R_CAN4_BodyZone_PS1/1 -> [R_CAN4_BodyZone_PS1]
  R_CAN4_PTG1/1 -> [R_CAN4_PTG1]
  R_CAN4_zGW_LINDr1/1 -> [R_CAN4_zGW_LINDr1]

== system SWC_CGW_type/run_SWC_CGW_sys/CGW/Sys_P_CAN6_CGW_GW6_CE100_0 ==
  R_CAN2_IVI1 : Inport
  R_CAN2_METER1 : Inport  Port=2
  R_CAN4_zGW_LINDr1 : Inport  Port=3
  bus_creator : BusCreator  Inputs=18  OutDataTypeStr=Bus: DT_CAN6_SG_CGW_GW6_CE100_0  NonVirtualBus=on
  bus_selector : BusSelector  OutputSignals=CAN2_IVI_Time_Day
  bus_selector1 : BusSelector  OutputSignals=CAN2_IVI_Time_Hour
  bus_selector10 : BusSelector  OutputSignals=CAN4_SWC2_L_ScrollUp_Sta
  bus_selector11 : BusSelector  OutputSignals=CAN4_SWC2_R_Customize_Sta
  bus_selector12 : BusSelector  OutputSignals=CAN4_SWC_ACC_Sta
  bus_selector13 : BusSelector  OutputSignals=CAN4_SWC_CANCEL_Sta
  bus_selector14 : BusSelector  OutputSignals=CAN4_SWC_Distance_Sta
  bus_selector15 : BusSelector  OutputSignals=CAN4_SWC_LKA_Sta
  bus_selector16 : BusSelector  OutputSignals=CAN4_SWC_Res_Up_Sta
  bus_selector17 : BusSelector  OutputSignals=CAN4_SWC_Set_down_Sta
  bus_selector2 : BusSelector  OutputSignals=CAN2_IVI_Time_Minute
  bus_selector3 : BusSelector  OutputSignals=CAN2_IVI_Time_Month
  bus_selector4 : BusSelector  OutputSignals=CAN2_IVI_Time_Second
  bus_selector5 : BusSelector  OutputSignals=CAN2_ODOMETER
  bus_selector6 : BusSelector  OutputSignals=CAN4_SWC2_L_ADAS_Sta
  bus_selector7 : BusSelector  OutputSignals=CAN4_SWC2_L_DriveMode_Sta
  bus_selector8 : BusSelector  OutputSignals=CAN4_SWC2_L_ScrollDown_Sta
  bus_selector9 : BusSelector  OutputSignals=CAN4_SWC2_L_ScrollPress_Sta
  P_CAN6_CGW_GW6_CE100_0 : Outport
  wires:
  bus_creator/1 -> P_CAN6_CGW_GW6_CE100_0/1
  bus_selector/1 -> bus_creator/1  "<CAN2_IVI_Time_Day>"
  [R_CAN2_IVI1] -> bus_selector/1
  bus_selector1/1 -> bus_creator/2  "<CAN2_IVI_Time_Hour>"
  [R_CAN2_IVI1] -> bus_selector1/1
  bus_selector2/1 -> bus_creator/3  "<CAN2_IVI_Time_Minute>"
  [R_CAN2_IVI1] -> bus_selector2/1
  bus_selector3/1 -> bus_creator/4  "<CAN2_IVI_Time_Month>"
  [R_CAN2_IVI1] -> bus_selector3/1
  bus_selector4/1 -> bus_creator/5  "<CAN2_IVI_Time_Second>"
  [R_CAN2_IVI1] -> bus_selector4/1
  bus_selector5/1 -> bus_creator/6  "<CAN2_ODOMETER>"
  [R_CAN2_METER1] -> bus_selector5/1
  bus_selector6/1 -> bus_creator/7  "<CAN4_SWC2_L_ADAS_Sta>"
  [R_CAN4_zGW_LINDr1] -> bus_selector6/1
  bus_selector7/1 -> bus_creator/8  "<CAN4_SWC2_L_DriveMode_Sta>"
  [R_CAN4_zGW_LINDr1] -> bus_selector7/1
  bus_selector8/1 -> bus_creator/9  "<CAN4_SWC2_L_ScrollDown_Sta>"
  [R_CAN4_zGW_LINDr1] -> bus_selector8/1
  bus_selector9/1 -> bus_creator/10  "<CAN4_SWC2_L_ScrollPress_Sta>"
  [R_CAN4_zGW_LINDr1] -> bus_selector9/1
  bus_selector10/1 -> bus_creator/11  "<CAN4_SWC2_L_ScrollUp_Sta>"
  [R_CAN4_zGW_LINDr1] -> bus_selector10/1
  bus_selector11/1 -> bus_creator/12  "<CAN4_SWC2_R_Customize_Sta>"
  [R_CAN4_zGW_LINDr1] -> bus_selector11/1
  bus_selector12/1 -> bus_creator/13  "<CAN4_SWC_ACC_Sta>"
  [R_CAN4_zGW_LINDr1] -> bus_selector12/1
  bus_selector13/1 -> bus_creator/14  "<CAN4_SWC_CANCEL_Sta>"
  [R_CAN4_zGW_LINDr1] -> bus_selector13/1
  bus_selector14/1 -> bus_creator/15  "<CAN4_SWC_Distance_Sta>"
  [R_CAN4_zGW_LINDr1] -> bus_selector14/1
  bus_selector15/1 -> bus_creator/16  "<CAN4_SWC_LKA_Sta>"
  [R_CAN4_zGW_LINDr1] -> bus_selector15/1
  bus_selector16/1 -> bus_creator/17  "<CAN4_SWC_Res_Up_Sta>"
  [R_CAN4_zGW_LINDr1] -> bus_selector16/1
  bus_selector17/1 -> bus_creator/18  "<CAN4_SWC_Set_down_Sta>"
  [R_CAN4_zGW_LINDr1] -> bus_selector17/1
  R_CAN2_IVI1/1 -> [R_CAN2_IVI1]
  R_CAN2_METER1/1 -> [R_CAN2_METER1]
  R_CAN4_zGW_LINDr1/1 -> [R_CAN4_zGW_LINDr1]

== system SWC_CGW_type/run_SWC_CGW_sys/CGW/Sys_P_CAN7_GW7_C100_0 ==
  R_CAN1_ESC1 : Inport
  bus_creator : BusCreator  Inputs=1  OutDataTypeStr=Bus: DT_CAN7_SG_GW7_C100_0  NonVirtualBus=on
  bus_selector : BusSelector  OutputSignals=CAN1_VehSpeed
  P_CAN7_GW7_C100_0 : Outport
  wires:
  bus_creator/1 -> P_CAN7_GW7_C100_0/1
  bus_selector/1 -> bus_creator/1  "<CAN1_VehSpeed>"
  [R_CAN1_ESC1] -> bus_selector/1
  R_CAN1_ESC1/1 -> [R_CAN1_ESC1]
